simulink model "Control_try_2"  (R2021a)
settings: Solver=VariableStepAuto  StartTime=0.0  StopTime=inf  RelTol=1e-3
undefined symbols (not defined in the file or in its folder): DiscIntNeverNeededParam
libraries: mobileRoboticsLib x25
(part 1 of 2)
settings Model: Creator=its_ghani  LastModifiedBy=2737767G

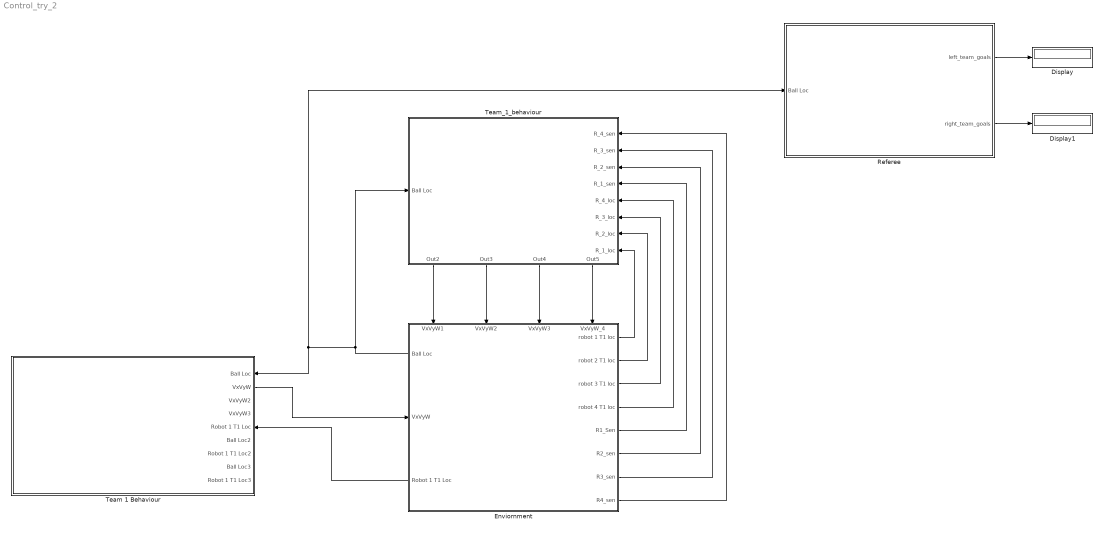
== system Control_try_2 ==
  Display : Display
  Display1 : Display
  Enviornment : Subsystem
      settings: PortSchema="{\"entries\":[{\"content\":{\"sides\":[{\"content\":{\"connectorIds\":[\"Out9\",\"In1\",\"Out10\"]},\"type\":\"ConnectorPlacement.EquallySpacedRectSide\",\"uuid\":\"bfc4f995-18bb-40a5-813e-439d500b4bf9\"},{\"content\":{\"connectorIds\":[\"Out1\",\"Out2\",\"Out3\",\"Out4\",\"Out5\",\"Out6\",\"Out7\",\"Out8\"],\"side\":\"RIGHT\"},\"type\":\"ConnectorPlacement.EquallySpacedRectSide\",\"uuid\":\"3fb6b8a6-16df-4a59-8ba5-6321e26d1fdd\"},{\"content\":{\"connectorIds\":[\"In2\",\"In3\",\"In4\",\"In5\"],\"side\":\"TOP\"},\"type\":\"ConnectorPlacement.EquallySpacedRectSide\",\"uuid\":\"a9e4cd1b-3afe-4395-99fa-15aef12a4070\"}]},\"type\":\"ConnectorPlacement.EquallySpacedConnector\",\"uuid\":\"a6ca697e-fe67-43ac-b669-91f3e6c836c9\"}],\"packageUris\":[\"http://schema.mathworks.com/mf0/Connector/R2020b\"],\"version\":\"1.0\"}"
  Referee : Subsystem
  Team 1 Behaviour : Subsystem
      settings: PortSchema="{\"entries\":[{\"content\":{\"sides\":[{\"content\":{\"connectorIds\":[]},\"type\":\"ConnectorPlacement.EquallySpacedRectSide\",\"uuid\":\"be901545-21b9-45e5-bac5-a8cb9027aef5\"},{\"content\":{\"connectorIds\":[\"In1\",\"Out1\",\"Out2\",\"Out3\",\"In2\",\"In3\",\"In4\",\"In5\",\"In6\"],\"side\":\"RIGHT\"},\"type\":\"ConnectorPlacement.EquallySpacedRectSide\",\"uuid\":\"b7c1eb84-2f14-4c7f-a74c-d56efbe0743e\"},{\"content\":{\"connectorIds\":[],\"side\":\"TOP\"},\"type\":\"ConnectorPlacement.EquallySpacedRectSide\",\"uuid\":\"aca41723-ed3f-4bd2-8fc1-457d075e3460\"}]},\"type\":\"ConnectorPlacement.EquallySpacedConnector\",\"uuid\":\"e10e22f1-c8f0-4dfc-85d2-4ba01528372d\"}],\"packageUris\":[\"http://schema.mathworks.com/mf0/Connector/R2020b\"],\"version\":\"1.0\"}"
  Team_1_behaviour : Subsystem
      settings: PortSchema="{\"entries\":[{\"content\":{\"sides\":[{\"content\":{\"connectorIds\":[\"In1\"]},\"type\":\"ConnectorPlacement.EquallySpacedRectSide\",\"uuid\":\"3d238569-03e8-47ba-93af-d09e13fdb2d4\"},{\"content\":{\"connectorIds\":[\"In2\",\"In3\",\"In4\",\"In5\",\"In6\",\"In7\",\"In8\",\"In9\"],\"side\":\"RIGHT\"},\"type\":\"ConnectorPlacement.EquallySpacedRectSide\",\"uuid\":\"12d8afb4-4727-4f82-8566-507ab080c6de\"},{\"content\":{\"connectorIds\":[],\"side\":\"TOP\"},\"type\":\"ConnectorPlacement.EquallySpacedRectSide\",\"uuid\":\"c52fa7ec-51b7-43be-84ca-6ce417c012c7\"},{\"content\":{\"connectorIds\":[\"Out1\",\"Out2\",\"Out3\",\"Out4\"],\"side\":\"BOTTOM\"},\"type\":\"ConnectorPlacement.EquallySpacedRectSide\",\"uuid\":\"1ba4ac49-8e90-4b3f-8374-c14756940453\"}]},\"type\":\"ConnectorPlacement.EquallySpacedConnector\",\"uuid\":\"883bb5df-d6b2-498f-94a4-3b94e28c6a8f\"}],\"packageUris\":[\"http://schema.mathworks.com/mf0/Connector/R2020b\"],\"version\":\"1.0\"}"
  wires:
  Enviornment/9(Ball Loc) -> Team_1_behaviour/1(Ball Loc), Referee/1(Ball Loc), Team 1 Behaviour/1(Ball Loc)
  Referee/2(right_team_goals) -> Display1/1
  Referee/1(left_team_goals) -> Display/1
  Team 1 Behaviour/1(VxVyW) -> Enviornment/1(VxVyW)
  Enviornment/10(Robot 1 T1 Loc) -> Team 1 Behaviour/2(Robot 1 T1 Loc)
  Team_1_behaviour/1(Out2) -> Enviornment/2(VxVyW1)
  Team_1_behaviour/2(Out3) -> Enviornment/3(VxVyW2)
  Team_1_behaviour/3(Out4) -> Enviornment/4(VxVyW3)
  Team_1_behaviour/4(Out5) -> Enviornment/5(VxVyW_4)
  Enviornment/1(robot 1 T1 loc) -> Team_1_behaviour/9(R_1_loc)
  Enviornment/2(robot 2 T1 loc) -> Team_1_behaviour/8(R_2_loc)
  Enviornment/3(robot 3 T1 loc) -> Team_1_behaviour/7(R_3_loc)
  Enviornment/4(robot 4 T1 loc) -> Team_1_behaviour/6(R_4_loc)
  Enviornment/5(R1_Sen) -> Team_1_behaviour/5(R_1_sen)
  Enviornment/6(R2_sen) -> Team_1_behaviour/4(R_2_sen)
  Enviornment/7(R3_sen) -> Team_1_behaviour/3(R_3_sen)
  Enviornment/8(R4_sen) -> Team_1_behaviour/2(R_4_sen)

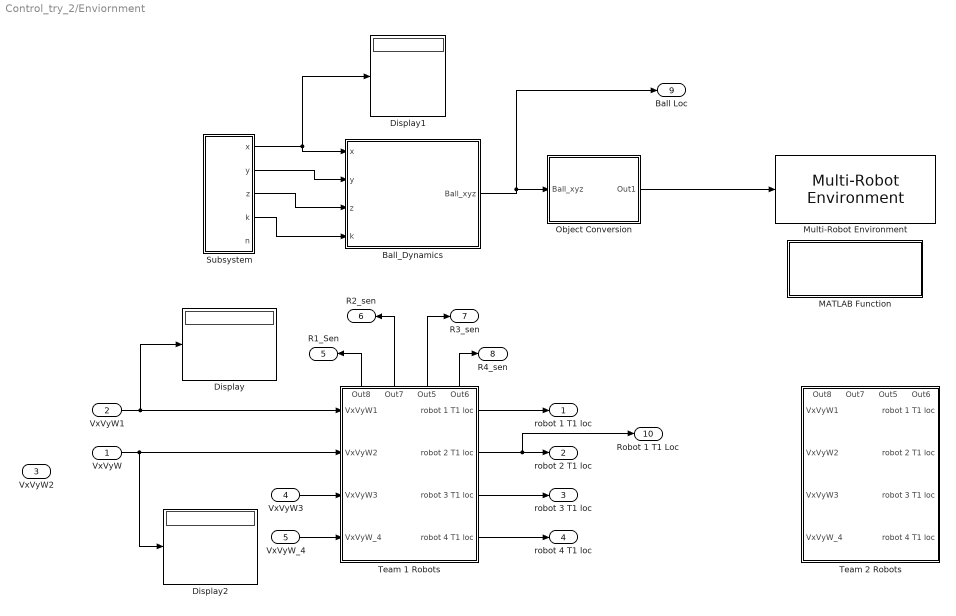
== system Control_try_2/Enviornment ==
  VxVyW : Inport
  VxVyW1 : Inport  Port=2
  VxVyW2 : Inport  Port=3
  VxVyW3 : Inport  Port=4
  VxVyW_4 : Inport  Port=5
  "\tTeam 1 Robots" : Subsystem
      settings: PortSchema="{\"entries\":[{\"content\":{\"sides\":[{\"content\":{\"connectorIds\":[\"In1\",\"In2\",\"In3\",\"In4\"]},\"type\":\"ConnectorPlacement.EquallySpacedRectSide\",\"uuid\":\"e759642f-fbca-4f1e-b212-daca2c4962f8\"},{\"content\":{\"connectorIds\":[\"Out1\",\"Out2\",\"Out3\",\"Out4\"],\"side\":\"RIGHT\"},\"type\":\"ConnectorPlacement.EquallySpacedRectSide\",\"uuid\":\"6e1699fa-b246-4758-836f-1d4c98857b70\"},{\"content\":{\"connectorIds\":[\"Out5\",\"Out6\",\"Out7\",\"Out8\"],\"side\":\"TOP\"},\"type\":\"ConnectorPlacement.EquallySpacedRectSide\",\"uuid\":\"c1cf0a96-808a-4241-9d01-181cc4ce2a4d\"},{\"content\":{\"connectorIds\":[],\"side\":\"BOTTOM\"},\"type\":\"ConnectorPlacement.EquallySpacedRectSide\",\"uuid\":\"1a7f648f-16d5-4a09-b479-d6590fa53252\"}]},\"type\":\"ConnectorPlacement.EquallySpacedConnector\",\"uuid\":\"5972ed04-ecdd-4117-bf5d-456318b5c4b8\"}],\"packageUris\":[\"http://schema.mathworks.com/mf0/Connector/R2020b\"],\"version\":\"1.0\"}"
  "\tTeam 2 Robots" : Subsystem
      settings: PortSchema="{\"entries\":[{\"content\":{\"sides\":[{\"content\":{\"connectorIds\":[\"In1\",\"In2\",\"In3\",\"In4\"]},\"type\":\"ConnectorPlacement.EquallySpacedRectSide\",\"uuid\":\"e759642f-fbca-4f1e-b212-daca2c4962f8\"},{\"content\":{\"connectorIds\":[\"Out1\",\"Out2\",\"Out3\",\"Out4\"],\"side\":\"RIGHT\"},\"type\":\"ConnectorPlacement.EquallySpacedRectSide\",\"uuid\":\"6e1699fa-b246-4758-836f-1d4c98857b70\"},{\"content\":{\"connectorIds\":[\"Out5\",\"Out6\",\"Out7\",\"Out8\"],\"side\":\"TOP\"},\"type\":\"ConnectorPlacement.EquallySpacedRectSide\",\"uuid\":\"c1cf0a96-808a-4241-9d01-181cc4ce2a4d\"},{\"content\":{\"connectorIds\":[],\"side\":\"BOTTOM\"},\"type\":\"ConnectorPlacement.EquallySpacedRectSide\",\"uuid\":\"1a7f648f-16d5-4a09-b479-d6590fa53252\"}]},\"type\":\"ConnectorPlacement.EquallySpacedConnector\",\"uuid\":\"5972ed04-ecdd-4117-bf5d-456318b5c4b8\"}],\"packageUris\":[\"http://schema.mathworks.com/mf0/Connector/R2020b\"],\"version\":\"1.0\"}"
  Ball_Dynamics : Subsystem
  Display : Display
  Display1 : Display
  Display2 : Display
  MATLAB Function : MATLAB Function  TreatAsAtomicUnit=on
  Multi-Robot Environment : mobileRoboticsLib/Environments/Multi-Robot Environment  numRobots=8  showWaypoints=off  showObjects=on  objectColors=[1 0 0;0 1 0;0 0 1]  objectMarkers='c'  showRobotIds=on  plotSensorLines=on
      settings: SourceProductName=Mobile Robotics Simulation Toolbox
  Object Conversion : Subsystem
  Subsystem : Subsystem
  robot 1 T1 loc : Outport
  robot 2 T1 loc : Outport  Port=2
  robot 3 T1 loc : Outport  Port=3
  robot 4 T1 loc : Outport  Port=4
  R1_Sen : Outport  Port=5
  R2_sen : Outport  Port=6
  R3_sen : Outport  Port=7
  R4_sen : Outport  Port=8
  Ball Loc : Outport  Port=9
  Robot 1 T1 Loc : Outport  Port=10
  wires:
  "\tTeam 1 Robots"/1(robot 1 T1 loc) -> robot 1 T1 loc/1
  Ball_Dynamics/1(Ball_xyz) -> Object Conversion/1(Ball_xyz), Ball Loc/1
  Object Conversion/1(Out1) -> Multi-Robot Environment/1
  "\tTeam 1 Robots"/2(robot 2 T1 loc) -> Robot 1 T1 Loc/1, robot 2 T1 loc/1
  "\tTeam 1 Robots"/3(robot 3 T1 loc) -> robot 3 T1 loc/1
  "\tTeam 1 Robots"/4(robot 4 T1 loc) -> robot 4 T1 loc/1
  VxVyW1/1 -> "\tTeam 1 Robots"/1(VxVyW1), Display/1
  VxVyW3/1 -> "\tTeam 1 Robots"/3(VxVyW3)
  VxVyW_4/1 -> "\tTeam 1 Robots"/4(VxVyW_4)
  "\tTeam 1 Robots"/5(Out8) -> R1_Sen/1
  "\tTeam 1 Robots"/6(Out7) -> R2_sen/1
  "\tTeam 1 Robots"/7(Out5) -> R3_sen/1
  "\tTeam 1 Robots"/8(Out6) -> R4_sen/1
  VxVyW/1 -> Display2/1, "\tTeam 1 Robots"/2(VxVyW2)
  Subsystem/1(x) -> Ball_Dynamics/1(x), Display1/1
  Subsystem/2(y) -> Ball_Dynamics/2(y)
  Subsystem/4(k) -> Ball_Dynamics/4(k)
  Subsystem/3(z) -> Ball_Dynamics/3(z)

== system Control_try_2/Referee ==
  Ball Loc : Inport
  Corner : Stateflow chart  TreatAsAtomicUnit=on
  Demux : Demux  Outputs=3
  Display2 : Display
  GOAL : Stateflow chart  TreatAsAtomicUnit=on
  Penelty : Stateflow chart  TreatAsAtomicUnit=on
  Throwin : Stateflow chart  TreatAsAtomicUnit=on
  left_team_goals : Outport
  right_team_goals : Outport  Port=2
  wires:
  Ball Loc/1 -> Display2/1, Demux/1
  Demux/1 -> Throwin/1(X), GOAL/1(X)
  Demux/2 -> Throwin/2(Y), GOAL/2(Y)
  Demux/3 -> GOAL/3(Z)
  GOAL/1(left_team_goal) -> left_team_goals/1
  GOAL/2(right_team_goal) -> right_team_goals/1

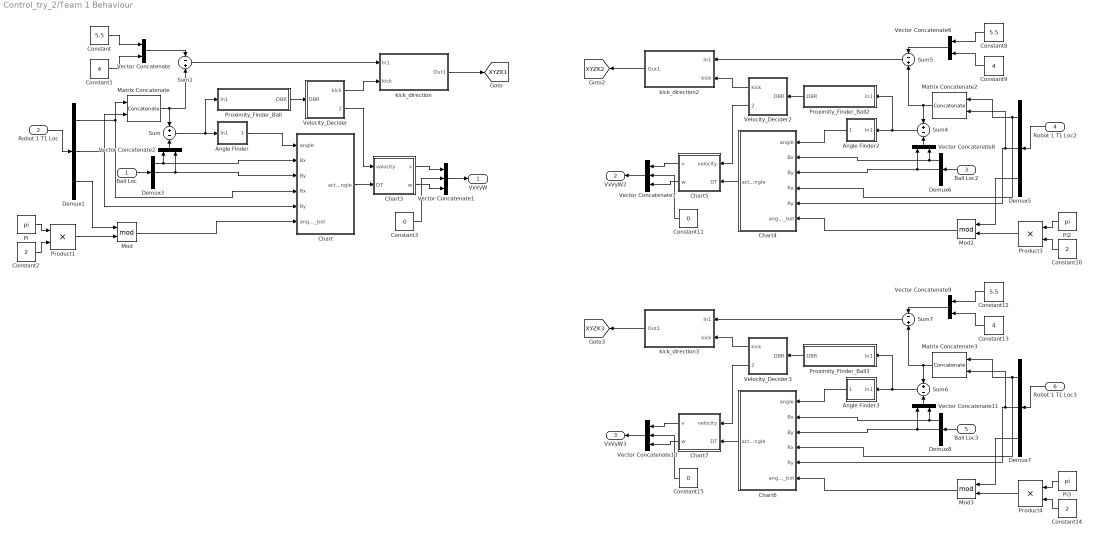
== system Control_try_2/Team 1 Behaviour ==
  Ball Loc : Inport
  Robot 1 T1 Loc : Inport  Port=2
  Ball Loc2 : Inport  Port=3
  Robot 1 T1 Loc2 : Inport  Port=4
  Ball Loc3 : Inport  Port=5
  Robot 1 T1 Loc3 : Inport  Port=6
  Angle Finder : Subsystem
  Angle Finder2 : Subsystem
  Angle Finder3 : Subsystem
  Chart : Stateflow chart  TreatAsAtomicUnit=on
      settings: PortSchema="{\"entries\":[{\"content\":{\"sides\":[{\"content\":{\"connectorIds\":[\"In5\",\"In1\",\"In2\",\"In3\",\"In4\",\"In6\"]},\"type\":\"ConnectorPlacement.EquallySpacedRectSide\",\"uuid\":\"cd25ea97-6441-4246-83f2-eec847899c89\"},{\"content\":{\"connectorIds\":[\"Out1\"],\"side\":\"RIGHT\"},\"type\":\"ConnectorPlacement.EquallySpacedRectSide\",\"uuid\":\"ef7d77a7-1549-4474-8b84-35bb8af5d0e7\"},{\"content\":{\"connectorIds\":[],\"side\":\"TOP\"},\"type\":\"ConnectorPlacement.EquallySpacedRectSide\",\"uuid\":\"0f0ce596-3061-42ac-890a-62bc4f21ac3e\"},{\"content\":{\"connectorIds\":[],\"side\":\"BOTTOM\"},\"type\":\"ConnectorPlacement.EquallySpacedRectSide\",\"uuid\":\"682b3de5-e999-4954-b7ff-f16ecbf9ea8f\"}]},\"type\":\"ConnectorPlacement.EquallySpacedConnector\",\"uuid\":\"15dca8e2-6a60-4a0d-80a5-3c295a61c828\"}],\"packageUris\":[\"http://schema.mathworks.com/mf0/Connector/R2020b\"],\"version\":\"1.0\"}"
  Chart3 : Stateflow chart  TreatAsAtomicUnit=on
  Chart4 : Stateflow chart  TreatAsAtomicUnit=on
      settings: PortSchema="{\"entries\":[{\"content\":{\"sides\":[{\"content\":{\"connectorIds\":[\"In5\",\"In1\",\"In2\",\"In3\",\"In4\",\"In6\"]},\"type\":\"ConnectorPlacement.EquallySpacedRectSide\",\"uuid\":\"cd25ea97-6441-4246-83f2-eec847899c89\"},{\"content\":{\"connectorIds\":[\"Out1\"],\"side\":\"RIGHT\"},\"type\":\"ConnectorPlacement.EquallySpacedRectSide\",\"uuid\":\"ef7d77a7-1549-4474-8b84-35bb8af5d0e7\"},{\"content\":{\"connectorIds\":[],\"side\":\"TOP\"},\"type\":\"ConnectorPlacement.EquallySpacedRectSide\",\"uuid\":\"0f0ce596-3061-42ac-890a-62bc4f21ac3e\"},{\"content\":{\"connectorIds\":[],\"side\":\"BOTTOM\"},\"type\":\"ConnectorPlacement.EquallySpacedRectSide\",\"uuid\":\"682b3de5-e999-4954-b7ff-f16ecbf9ea8f\"}]},\"type\":\"ConnectorPlacement.EquallySpacedConnector\",\"uuid\":\"15dca8e2-6a60-4a0d-80a5-3c295a61c828\"}],\"packageUris\":[\"http://schema.mathworks.com/mf0/Connector/R2020b\"],\"version\":\"1.0\"}"
  Chart5 : Stateflow chart  TreatAsAtomicUnit=on
  Chart6 : Stateflow chart  TreatAsAtomicUnit=on
      settings: PortSchema="{\"entries\":[{\"content\":{\"sides\":[{\"content\":{\"connectorIds\":[\"In5\",\"In1\",\"In2\",\"In3\",\"In4\",\"In6\"]},\"type\":\"ConnectorPlacement.EquallySpacedRectSide\",\"uuid\":\"cd25ea97-6441-4246-83f2-eec847899c89\"},{\"content\":{\"connectorIds\":[\"Out1\"],\"side\":\"RIGHT\"},\"type\":\"ConnectorPlacement.EquallySpacedRectSide\",\"uuid\":\"ef7d77a7-1549-4474-8b84-35bb8af5d0e7\"},{\"content\":{\"connectorIds\":[],\"side\":\"TOP\"},\"type\":\"ConnectorPlacement.EquallySpacedRectSide\",\"uuid\":\"0f0ce596-3061-42ac-890a-62bc4f21ac3e\"},{\"content\":{\"connectorIds\":[],\"side\":\"BOTTOM\"},\"type\":\"ConnectorPlacement.EquallySpacedRectSide\",\"uuid\":\"682b3de5-e999-4954-b7ff-f16ecbf9ea8f\"}]},\"type\":\"ConnectorPlacement.EquallySpacedConnector\",\"uuid\":\"15dca8e2-6a60-4a0d-80a5-3c295a61c828\"}],\"packageUris\":[\"http://schema.mathworks.com/mf0/Connector/R2020b\"],\"version\":\"1.0\"}"
  Chart7 : Stateflow chart  TreatAsAtomicUnit=on
  Constant : Constant  Value=5.5
  Constant1 : Constant  Value=4
  Constant10 : Constant  Value=2
  Constant11 : Constant  Value=0
  Constant12 : Constant  Value=5.5
  Constant13 : Constant  Value=4
  Constant14 : Constant  Value=2
  Constant15 : Constant  Value=0
  Constant2 : Constant  Value=2
  Constant3 : Constant  Value=0
  Constant8 : Constant  Value=5.5
  Constant9 : Constant  Value=4
  Demux{1,3,5..8} (6 alike) : Demux  Outputs=3
  Matrix Concatenate : Concatenate  Mode=Multidimensional array  ConcatenateDimension=2
  Matrix Concatenate2 : Concatenate  Mode=Multidimensional array  ConcatenateDimension=2
  Matrix Concatenate3 : Concatenate  Mode=Multidimensional array  ConcatenateDimension=2
  Mod : Math  Operator=mod  SaturateOnIntegerOverflow=on
  Mod2 : Math  Operator=mod  SaturateOnIntegerOverflow=on
  Mod3 : Math  Operator=mod  SaturateOnIntegerOverflow=on
  Pi : Constant  Value=pi  OutDataTypeStr=Inherit: Inherit via back propagation
  Pi2 : Constant  Value=pi  OutDataTypeStr=Inherit: Inherit via back propagation
  Pi3 : Constant  Value=pi  OutDataTypeStr=Inherit: Inherit via back propagation
  Product1 : Product
  Product3 : Product
  Product4 : Product
  Proximity_Finder_Ball : Subsystem
  Proximity_Finder_Ball2 : Subsystem
  Proximity_Finder_Ball3 : Subsystem
  Sum : Sum  Inputs=+-
  Sum1 : Sum  Inputs=-+
  Sum4 : Sum  Inputs=+-
  Sum5 : Sum  Inputs=-+
  Sum6 : Sum  Inputs=+-
  Sum7 : Sum  Inputs=-+
  Vector Concatenate{,2,6,8..9,11} (6 alike) : Concatenate
  Vector Concatenate1 : Concatenate  NumInputs=3
  Vector Concatenate10 : Concatenate  NumInputs=3
  Vector Concatenate7 : Concatenate  NumInputs=3
  Velocity_Decider : Stateflow chart  TreatAsAtomicUnit=on
  Velocity_Decider2 : Stateflow chart  TreatAsAtomicUnit=on
  Velocity_Decider3 : Stateflow chart  TreatAsAtomicUnit=on
  kick_direction : Subsystem
  kick_direction2 : Subsystem
  kick_direction3 : Subsystem
  VxVyW : Outport
  VxVyW2 : Outport  Port=2
  VxVyW3 : Outport  Port=3
  tag scope: XYZK1=global, XYZK2=global, XYZK3=global
  wires:
  Ball Loc/1 -> Demux3/1
  Sum/1 -> Proximity_Finder_Ball/1(In1), Angle Finder/1(In1)
  Robot 1 T1 Loc/1 -> Demux1/1
  Demux1/1 -> Matrix Concatenate/1, Chart/3(Rx)
  Demux1/2 -> Matrix Concatenate/2, Chart/4(Ry)
  Matrix Concatenate/1 -> Sum1/2, Sum/1
  Demux3/2 -> Vector Concatenate2/2, Chart/2(By)
  Demux3/1 -> Vector Concatenate2/1, Chart/1(Bx)
  Demux1/3 -> Mod/1
  Pi/1 -> Product1/1
  Constant2/1 -> Product1/2
  Product1/1 -> Mod/2
  Chart/1(actual_angle) -> Chart3/2(DT)
  Mod/1 -> Chart/6(angle_bot)
  Angle Finder/1(angle) -> Chart/5(angle)
  Proximity_Finder_Ball/1(DBR) -> Velocity_Decider/1(DBR)
  Velocity_Decider/2(velocity) -> Chart3/1(velocity)
  Constant/1 -> Vector Concatenate/1
  Constant1/1 -> Vector Concatenate/2
  Vector Concatenate/1 -> Sum1/1
  Sum1/1 -> kick_direction/1(In1)
  Velocity_Decider/1(kick) -> kick_direction/2(kick)
  kick_direction/1(Out1) -> [XYZK1]
  Chart3/1(v) -> Vector Concatenate1/1
  Chart3/2(w) -> Vector Concatenate1/3
  Constant3/1 -> Vector Concatenate1/2
  Vector Concatenate1/1 -> VxVyW/1
  Vector Concatenate2/1 -> Sum/2
  Constant11/1 -> Vector Concatenate7/2
  Pi2/1 -> Product3/1
  Chart5/1(v) -> Vector Concatenate7/1
  Vector Concatenate8/1 -> Sum4/2
  Velocity_Decider2/1(kick) -> kick_direction2/2(kick)
  Sum5/1 -> kick_direction2/1(In1)
  Velocity_Decider2/2(velocity) -> Chart5/1(velocity)
  Constant8/1 -> Vector Concatenate6/1
  Vector Concatenate7/1 -> VxVyW2/1
  Vector Concatenate6/1 -> Sum5/1
  Product3/1 -> Mod2/2
  Chart5/2(w) -> Vector Concatenate7/3
  Sum4/1 -> Proximity_Finder_Ball2/1(In1), Angle Finder2/1(In1)
  Constant10/1 -> Product3/2
  kick_direction2/1(Out1) -> [XYZK2]
  Demux6/2 -> Vector Concatenate8/2, Chart4/2(By)
  Chart4/1(actual_angle) -> Chart5/2(DT)
  Constant9/1 -> Vector Concatenate6/2
  Matrix Concatenate2/1 -> Sum5/2, Sum4/1
  Mod2/1 -> Chart4/6(angle_bot)
  Proximity_Finder_Ball2/1(DBR) -> Velocity_Decider2/1(DBR)
  Robot 1 T1 Loc2/1 -> Demux5/1
  Demux5/2 -> Matrix Concatenate2/2, Chart4/4(Ry)
  Demux5/1 -> Matrix Concatenate2/1, Chart4/3(Rx)
  Angle Finder2/1(angle) -> Chart4/5(angle)
  Demux6/1 -> Vector Concatenate8/1, Chart4/1(Bx)
  Ball Loc2/1 -> Demux6/1
  Demux5/3 -> Mod2/1
  Constant15/1 -> Vector Concatenate10/2
  Pi3/1 -> Product4/1
  Chart7/1(v) -> Vector Concatenate10/1
  Vector Concatenate11/1 -> Sum6/2
  Velocity_Decider3/1(kick) -> kick_direction3/2(kick)
  Sum7/1 -> kick_direction3/1(In1)
  Velocity_Decider3/2(velocity) -> Chart7/1(velocity)
  Constant12/1 -> Vector Concatenate9/1
  Vector Concatenate10/1 -> VxVyW3/1
  Vector Concatenate9/1 -> Sum7/1
  Product4/1 -> Mod3/2
  Chart7/2(w) -> Vector Concatenate10/3
  Sum6/1 -> Proximity_Finder_Ball3/1(In1), Angle Finder3/1(In1)
  Constant14/1 -> Product4/2
  kick_direction3/1(Out1) -> [XYZK3]
  Demux8/2 -> Vector Concatenate11/2, Chart6/2(By)
  Chart6/1(actual_angle) -> Chart7/2(DT)
  Constant13/1 -> Vector Concatenate9/2
  Matrix Concatenate3/1 -> Sum7/2, Sum6/1
  Mod3/1 -> Chart6/6(angle_bot)
  Proximity_Finder_Ball3/1(DBR) -> Velocity_Decider3/1(DBR)
  Robot 1 T1 Loc3/1 -> Demux7/1
  Demux7/2 -> Matrix Concatenate3/2, Chart6/4(Ry)
  Demux7/1 -> Matrix Concatenate3/1, Chart6/3(Rx)
  Angle Finder3/1(angle) -> Chart6/5(angle)
  Demux8/1 -> Vector Concatenate11/1, Chart6/1(Bx)
  Ball Loc3/1 -> Demux8/1
  Demux7/3 -> Mod3/1

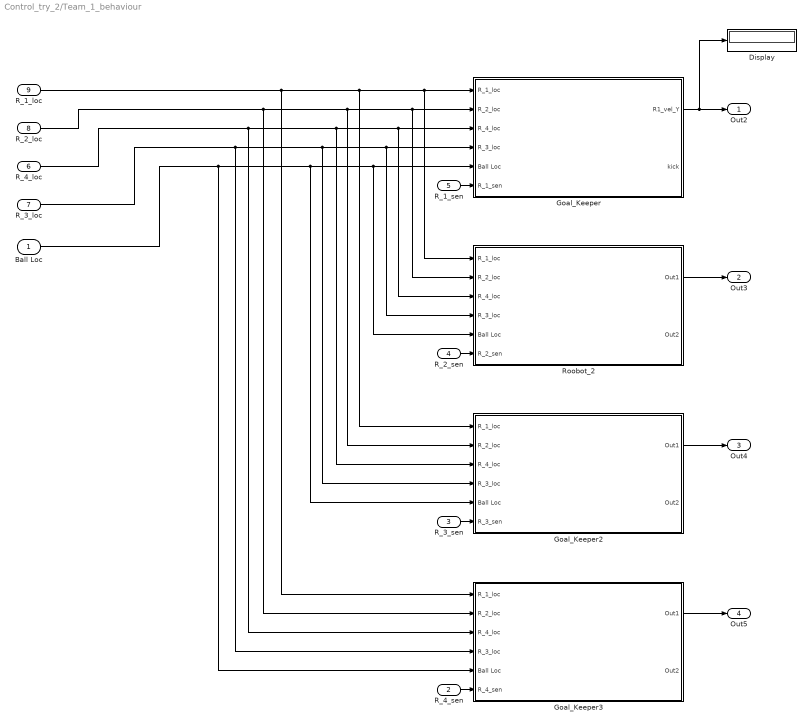
== system Control_try_2/Team_1_behaviour ==
  Ball Loc : Inport
  R_4_sen : Inport  Port=2
  R_3_sen : Inport  Port=3
  R_2_sen : Inport  Port=4
  R_1_sen : Inport  Port=5
  R_4_loc : Inport  Port=6
  R_3_loc : Inport  Port=7
  R_2_loc : Inport  Port=8
  R_1_loc : Inport  Port=9
  Display : Display
  Goal_Keeper : Subsystem
  Goal_Keeper2 : Subsystem
  Goal_Keeper3 : Subsystem
  Roobot_2 : Subsystem
  Out2 : Outport
  Out3 : Outport  Port=2
  Out4 : Outport  Port=3
  Out5 : Outport  Port=4
  wires:
  Goal_Keeper/1(R1_vel_Y) -> Display/1, Out2/1
  R_1_sen/1 -> Goal_Keeper/6(R_1_sen)
  R_1_loc/1 -> Goal_Keeper3/1(R_1_loc), Goal_Keeper2/1(R_1_loc), Roobot_2/1(R_1_loc), Goal_Keeper/1(R_1_loc)
  R_2_loc/1 -> Goal_Keeper3/2(R_2_loc), Goal_Keeper2/2(R_2_loc), Roobot_2/2(R_2_loc), Goal_Keeper/2(R_2_loc)
  R_4_loc/1 -> Goal_Keeper3/3(R_4_loc), Goal_Keeper2/3(R_4_loc), Roobot_2/3(R_4_loc), Goal_Keeper/3(R_4_loc)
  R_3_loc/1 -> Goal_Keeper3/4(R_3_loc), Goal_Keeper2/4(R_3_loc), Roobot_2/4(R_3_loc), Goal_Keeper/4(R_3_loc)
  Ball Loc/1 -> Goal_Keeper3/5(Ball Loc), Goal_Keeper2/5(Ball Loc), Roobot_2/5(Ball Loc), Goal_Keeper/5(Ball Loc)
  R_2_sen/1 -> Roobot_2/6(R_2_sen)
  R_3_sen/1 -> Goal_Keeper2/6(R_3_sen)
  R_4_sen/1 -> Goal_Keeper3/6(R_4_sen)
  Roobot_2/1(Out1) -> Out3/1
  Goal_Keeper2/1(Out1) -> Out4/1
  Goal_Keeper3/1(Out1) -> Out5/1

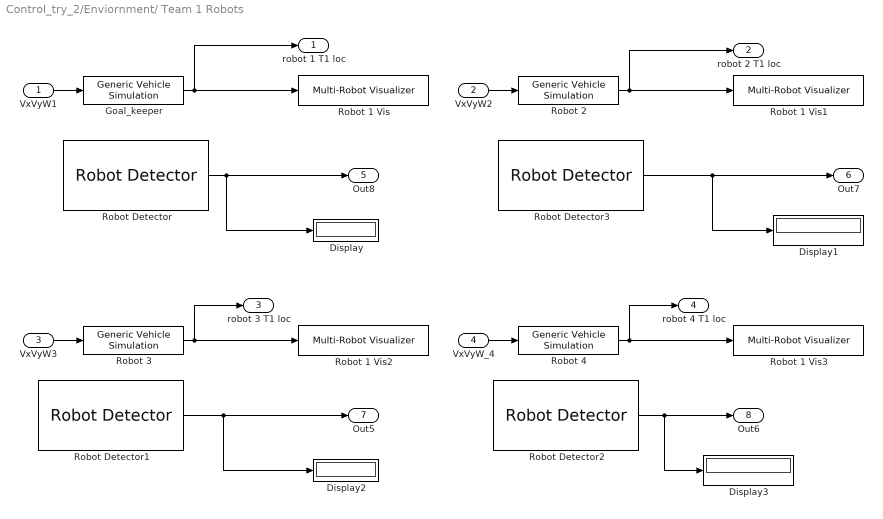
== system Control_try_2/Enviornment/	Team 1 Robots ==
  VxVyW1 : Inport
  VxVyW2 : Inport  Port=2
  VxVyW3 : Inport  Port=3
  VxVyW_4 : Inport  Port=4
  Display{,1..3} (4 alike) : Display
  Goal_keeper : mobileRoboticsLib/Utilities/Generic Vehicle Simulation  initX=1.5  initY=4  initAngle=0  Ts=0.05
      settings: SourceProductName=Mobile Robotics Simulation Toolbox
  Robot 1 Vis : mobileRoboticsLib/Environments/Multi-Robot Visualizer  idx=1  radius=0.5  robotColor=[0 0 1]  showTraj=on  hasLidar=off  sensorOffset=[0,0]  scanAngles=[-pi/4, 0, pi/4]  maxNumScans=0  hasObjDetector=off  objDetectorOffset=[0,0]  objDetectorAngle=0  objDetectorFOV=pi/3  objDetectorMaxRange=5  hasRobotDetector=off  robotDetectorOffset=[0,0]  robotDetectorAngle=0  robotDetectorFOV=pi/3  robotDetectorMaxRange=5  robotDetectorNumDetections=0
      settings: SourceProductName=Mobile Robotics Simulation Toolbox
  Robot 1 Vis1 : mobileRoboticsLib/Environments/Multi-Robot Visualizer  idx=2  radius=0.5  robotColor=[0 0 1]  showTraj=on  hasLidar=off  sensorOffset=[0,0]  scanAngles=[-pi/4, 0, pi/4]  maxNumScans=0  hasObjDetector=off  objDetectorOffset=[0,0]  objDetectorAngle=0  objDetectorFOV=pi/3  objDetectorMaxRange=5  hasRobotDetector=off  robotDetectorOffset=[0,0]  robotDetectorAngle=0  robotDetectorFOV=pi/3  robotDetectorMaxRange=5  robotDetectorNumDetections=0
      settings: SourceProductName=Mobile Robotics Simulation Toolbox
  Robot 1 Vis2 : mobileRoboticsLib/Environments/Multi-Robot Visualizer  idx=3  radius=0.5  robotColor=[0 0 1]  showTraj=on  hasLidar=off  sensorOffset=[0,0]  scanAngles=[-pi/4, 0, pi/4]  maxNumScans=0  hasObjDetector=off  objDetectorOffset=[0,0]  objDetectorAngle=0  objDetectorFOV=pi/3  objDetectorMaxRange=5  hasRobotDetector=off  robotDetectorOffset=[0,0]  robotDetectorAngle=0  robotDetectorFOV=pi/3  robotDetectorMaxRange=5  robotDetectorNumDetections=0
      settings: SourceProductName=Mobile Robotics Simulation Toolbox
  Robot 1 Vis3 : mobileRoboticsLib/Environments/Multi-Robot Visualizer  idx=4  radius=0.5  robotColor=[0 0 1]  showTraj=on  hasLidar=off  sensorOffset=[0,0]  scanAngles=[-pi/4, 0, pi/4]  maxNumScans=0  hasObjDetector=off  objDetectorOffset=[0,0]  objDetectorAngle=0  objDetectorFOV=pi/3  objDetectorMaxRange=5  hasRobotDetector=off  robotDetectorOffset=[0,0]  robotDetectorAngle=0  robotDetectorFOV=pi/3  robotDetectorMaxRange=5  robotDetectorNumDetections=0
      settings: SourceProductName=Mobile Robotics Simulation Toolbox
  Robot 2 : mobileRoboticsLib/Utilities/Generic Vehicle Simulation  initX=3.25  initY=2.5  initAngle=0  Ts=0.05
      settings: SourceProductName=Mobile Robotics Simulation Toolbox
  Robot 3 : mobileRoboticsLib/Utilities/Generic Vehicle Simulation  initX=3.25  initY=5.5  initAngle=0  Ts=0.05
      settings: SourceProductName=Mobile Robotics Simulation Toolbox
  Robot 4 : mobileRoboticsLib/Utilities/Generic Vehicle Simulation  initX=5.25  initY=4.25  initAngle=0  Ts=0.05
      settings: SourceProductName=Mobile Robotics Simulation Toolbox
  Robot Detector : mobileRoboticsLib/Environments/Robot Detector  mapName=map  robotIdx=1  sensorOffset=[ 0, 0 ]  sensorAngle=0  sensorFOV=pi/3  maxRange=3  maxDetections=7  sampleTime=0.1
      settings: SourceProductName=Mobile Robotics Simulation Toolbox
  Robot Detector1 : mobileRoboticsLib/Environments/Robot Detector  mapName=map  robotIdx=3  sensorOffset=[ 0, 0 ]  sensorAngle=0  sensorFOV=pi/3  maxRange=1.5  maxDetections=7  sampleTime=0.1
      settings: SourceProductName=Mobile Robotics Simulation Toolbox
  Robot Detector2 : mobileRoboticsLib/Environments/Robot Detector  mapName=map  robotIdx=4  sensorOffset=[ 0, 0 ]  sensorAngle=0  sensorFOV=pi/3  maxRange=1.5  maxDetections=7  sampleTime=0.1
      settings: SourceProductName=Mobile Robotics Simulation Toolbox
  Robot Detector3 : mobileRoboticsLib/Environments/Robot Detector  mapName=map  robotIdx=2  sensorOffset=[ 0, 0 ]  sensorAngle=0  sensorFOV=pi/3  maxRange=1.5  maxDetections=7  sampleTime=0.1
      settings: SourceProductName=Mobile Robotics Simulation Toolbox
  robot 1 T1 loc : Outport
  robot 2 T1 loc : Outport  Port=2
  robot 3 T1 loc : Outport  Port=3
  robot 4 T1 loc : Outport  Port=4
  Out8 : Outport  Port=5
  Out7 : Outport  Port=6
  Out5 : Outport  Port=7
  Out6 : Outport  Port=8
  wires:
  Goal_keeper/1 -> robot 1 T1 loc/1, Robot 1 Vis/1
  VxVyW1/1 -> Goal_keeper/1
  VxVyW2/1 -> Robot 2/1
  Robot 2/1 -> robot 2 T1 loc/1, Robot 1 Vis1/1
  Robot 3/1 -> Robot 1 Vis2/1, robot 3 T1 loc/1
  VxVyW3/1 -> Robot 3/1
  VxVyW_4/1 -> Robot 4/1
  Robot 4/1 -> robot 4 T1 loc/1, Robot 1 Vis3/1
  Robot Detector3/1 -> Out7/1, Display1/1
  Robot Detector1/1 -> Out5/1, Display2/1
  Robot Detector2/1 -> Out6/1, Display3/1
  Robot Detector/1 -> Display/1, Out8/1

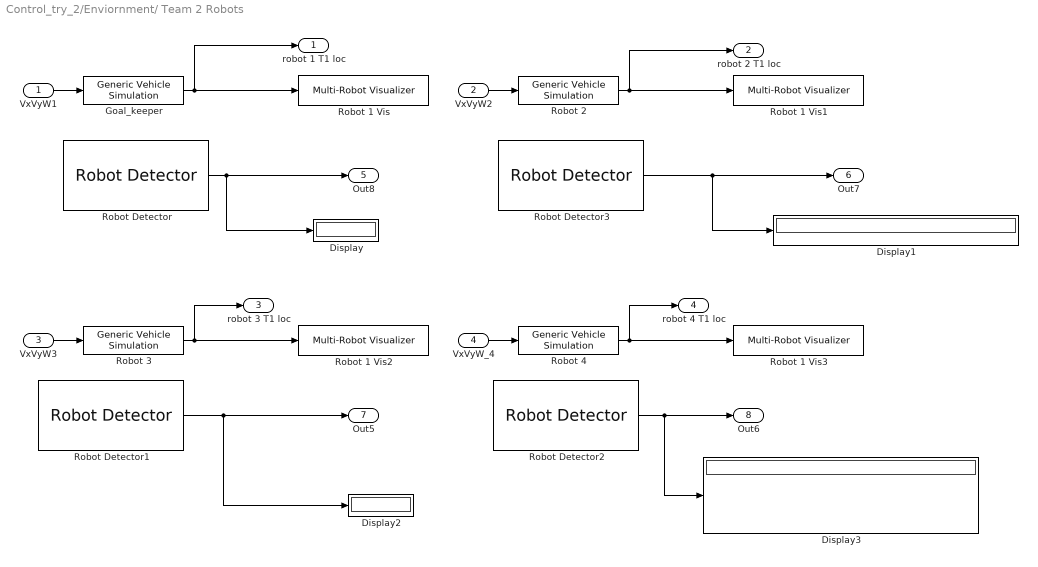
== system Control_try_2/Enviornment/	Team 2 Robots ==
  VxVyW1 : Inport
  VxVyW2 : Inport  Port=2
  VxVyW3 : Inport  Port=3
  VxVyW_4 : Inport  Port=4
  Display{,1..3} (4 alike) : Display
  Goal_keeper : mobileRoboticsLib/Utilities/Generic Vehicle Simulation  initX=9.5  initY=4  initAngle=pi  Ts=0.05
      settings: SourceProductName=Mobile Robotics Simulation Toolbox
  Robot 1 Vis : mobileRoboticsLib/Environments/Multi-Robot Visualizer  idx=5  radius=0.5  robotColor=[1 0 0]  showTraj=on  hasLidar=off  sensorOffset=[0,0]  scanAngles=[-pi/4, 0, pi/4]  maxNumScans=0  hasObjDetector=off  objDetectorOffset=[0,0]  objDetectorAngle=0  objDetectorFOV=pi/3  objDetectorMaxRange=5  hasRobotDetector=off  robotDetectorOffset=[0,0]  robotDetectorAngle=0  robotDetectorFOV=pi/3  robotDetectorMaxRange=5  robotDetectorNumDetections=0
      settings: SourceProductName=Mobile Robotics Simulation Toolbox
  Robot 1 Vis1 : mobileRoboticsLib/Environments/Multi-Robot Visualizer  idx=6  radius=0.5  robotColor=[0.1 1 1]  showTraj=on  hasLidar=off  sensorOffset=[0,0]  scanAngles=[-pi/4, 0, pi/4]  maxNumScans=0  hasObjDetector=off  objDetectorOffset=[0,0]  objDetectorAngle=0  objDetectorFOV=pi/3  objDetectorMaxRange=5  hasRobotDetector=off  robotDetectorOffset=[0,0]  robotDetectorAngle=0  robotDetectorFOV=pi/3  robotDetectorMaxRange=5  robotDetectorNumDetections=0
      settings: SourceProductName=Mobile Robotics Simulation Toolbox
  Robot 1 Vis2 : mobileRoboticsLib/Environments/Multi-Robot Visualizer  idx=7  radius=0.5  robotColor=[0 1 1]  showTraj=on  hasLidar=off  sensorOffset=[0,0]  scanAngles=[-pi/4, 0, pi/4]  maxNumScans=0  hasObjDetector=off  objDetectorOffset=[0,0]  objDetectorAngle=0  objDetectorFOV=pi/3  objDetectorMaxRange=5  hasRobotDetector=off  robotDetectorOffset=[0,0]  robotDetectorAngle=0  robotDetectorFOV=pi/3  robotDetectorMaxRange=5  robotDetectorNumDetections=0
      settings: SourceProductName=Mobile Robotics Simulation Toolbox
  Robot 1 Vis3 : mobileRoboticsLib/Environments/Multi-Robot Visualizer  idx=8  radius=0.5  robotColor=[0 1 1]  showTraj=on  hasLidar=off  sensorOffset=[0,0]  scanAngles=[-pi/4, 0, pi/4]  maxNumScans=0  hasObjDetector=off  objDetectorOffset=[0,0]  objDetectorAngle=0  objDetectorFOV=pi/3  objDetectorMaxRange=5  hasRobotDetector=off  robotDetectorOffset=[0,0]  robotDetectorAngle=0  robotDetectorFOV=pi/3  robotDetectorMaxRange=5  robotDetectorNumDetections=0
      settings: SourceProductName=Mobile Robotics Simulation Toolbox
  Robot 2 : mobileRoboticsLib/Utilities/Generic Vehicle Simulation  initX=3.5  initY=4  initAngle=pi  Ts=0.05
      settings: SourceProductName=Mobile Robotics Simulation Toolbox
  Robot 3 : mobileRoboticsLib/Utilities/Generic Vehicle Simulation  initX=3.5  initY=3  initAngle=pi  Ts=0.05
      settings: SourceProductName=Mobile Robotics Simulation Toolbox
  Robot 4 : mobileRoboticsLib/Utilities/Generic Vehicle Simulation  initX=7.75  initY=2.5  initAngle=pi  Ts=0.05
      settings: SourceProductName=Mobile Robotics Simulation Toolbox
  Robot Detector : mobileRoboticsLib/Environments/Robot Detector  mapName=map  robotIdx=5  sensorOffset=[ 0, 0 ]  sensorAngle=0  sensorFOV=pi/3  maxRange=1.5  maxDetections=7  sampleTime=0.1
      settings: SourceProductName=Mobile Robotics Simulation Toolbox
  Robot Detector1 : mobileRoboticsLib/Environments/Robot Detector  mapName=map  robotIdx=7  sensorOffset=[ 0, 0 ]  sensorAngle=0  sensorFOV=pi/3  maxRange=1.5  maxDetections=7  sampleTime=0.1
      settings: SourceProductName=Mobile Robotics Simulation Toolbox
  Robot Detector2 : mobileRoboticsLib/Environments/Robot Detector  mapName=map  robotIdx=8  sensorOffset=[ 0, 0 ]  sensorAngle=0  sensorFOV=pi/3  maxRange=1.5  maxDetections=7  sampleTime=0.1
      settings: SourceProductName=Mobile Robotics Simulation Toolbox
  Robot Detector3 : mobileRoboticsLib/Environments/Robot Detector  mapName=map  robotIdx=6  sensorOffset=[ 0, 0 ]  sensorAngle=0  sensorFOV=pi/3  maxRange=1.5  maxDetections=7  sampleTime=0.1
      settings: SourceProductName=Mobile Robotics Simulation Toolbox
  robot 1 T1 loc : Outport
  robot 2 T1 loc : Outport  Port=2
  robot 3 T1 loc : Outport  Port=3
  robot 4 T1 loc : Outport  Port=4
  Out8 : Outport  Port=5
  Out7 : Outport  Port=6
  Out5 : Outport  Port=7
  Out6 : Outport  Port=8
  wires:
  Goal_keeper/1 -> robot 1 T1 loc/1, Robot 1 Vis/1
  VxVyW1/1 -> Goal_keeper/1
  VxVyW2/1 -> Robot 2/1
  Robot 2/1 -> robot 2 T1 loc/1, Robot 1 Vis1/1
  Robot 3/1 -> Robot 1 Vis2/1, robot 3 T1 loc/1
  VxVyW3/1 -> Robot 3/1
  VxVyW_4/1 -> Robot 4/1
  Robot 4/1 -> robot 4 T1 loc/1, Robot 1 Vis3/1
  Robot Detector3/1 -> Out7/1, Display1/1
  Robot Detector1/1 -> Out5/1, Display2/1
  Robot Detector2/1 -> Out6/1, Display3/1
  Robot Detector/1 -> Display/1, Out8/1

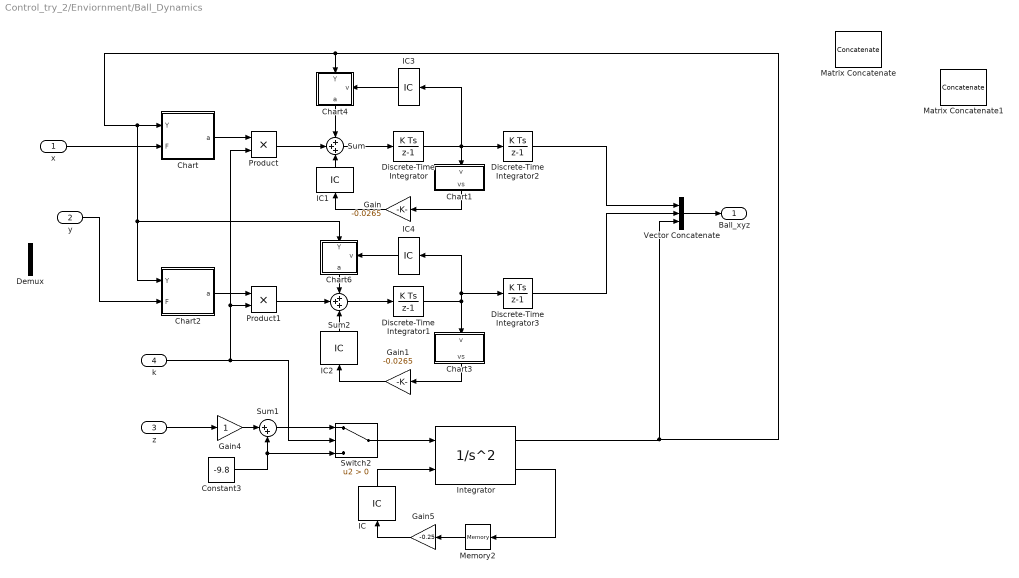
== system Control_try_2/Enviornment/Ball_Dynamics ==
  x : Inport
  y : Inport  Port=2
  z : Inport  Port=3
  k : Inport  Port=4
  Chart : Stateflow chart  TreatAsAtomicUnit=on
  Chart1 : Stateflow chart  TreatAsAtomicUnit=on
      settings: PortSchema="{\"entries\":[{\"content\":{\"sides\":[{\"content\":{\"connectorIds\":[]},\"type\":\"ConnectorPlacement.EquallySpacedRectSide\",\"uuid\":\"edcb69b6-c92b-474e-86d7-1e52c2e82b28\"},{\"content\":{\"connectorIds\":[],\"side\":\"RIGHT\"},\"type\":\"ConnectorPlacement.EquallySpacedRectSide\",\"uuid\":\"df9771e4-6870-4305-9c84-3f71fcb76e6b\"},{\"content\":{\"connectorIds\":[\"In1\"],\"side\":\"TOP\"},\"type\":\"ConnectorPlacement.EquallySpacedRectSide\",\"uuid\":\"56b80241-156d-4669-9174-884a577f2013\"},{\"content\":{\"connectorIds\":[\"Out1\"],\"side\":\"BOTTOM\"},\"type\":\"ConnectorPlacement.EquallySpacedRectSide\",\"uuid\":\"179af6a7-cab5-4faa-a562-268e2d2e4d3e\"}]},\"type\":\"ConnectorPlacement.EquallySpacedConnector\",\"uuid\":\"707001f1-02b8-4f5e-ba3f-f155c99072e5\"}],\"packageUris\":[\"http://schema.mathworks.com/mf0/Connector/R2020b\"],\"version\":\"1.0\"}"
  Chart2 : Stateflow chart  TreatAsAtomicUnit=on
  Chart3 : Stateflow chart  TreatAsAtomicUnit=on
      settings: PortSchema="{\"entries\":[{\"content\":{\"sides\":[{\"content\":{\"connectorIds\":[]},\"type\":\"ConnectorPlacement.EquallySpacedRectSide\",\"uuid\":\"edcb69b6-c92b-474e-86d7-1e52c2e82b28\"},{\"content\":{\"connectorIds\":[],\"side\":\"RIGHT\"},\"type\":\"ConnectorPlacement.EquallySpacedRectSide\",\"uuid\":\"df9771e4-6870-4305-9c84-3f71fcb76e6b\"},{\"content\":{\"connectorIds\":[\"In1\"],\"side\":\"TOP\"},\"type\":\"ConnectorPlacement.EquallySpacedRectSide\",\"uuid\":\"56b80241-156d-4669-9174-884a577f2013\"},{\"content\":{\"connectorIds\":[\"Out1\"],\"side\":\"BOTTOM\"},\"type\":\"ConnectorPlacement.EquallySpacedRectSide\",\"uuid\":\"179af6a7-cab5-4faa-a562-268e2d2e4d3e\"}]},\"type\":\"ConnectorPlacement.EquallySpacedConnector\",\"uuid\":\"707001f1-02b8-4f5e-ba3f-f155c99072e5\"}],\"packageUris\":[\"http://schema.mathworks.com/mf0/Connector/R2020b\"],\"version\":\"1.0\"}"
  Chart4 : Stateflow chart  TreatAsAtomicUnit=on
      settings: PortSchema="{\"entries\":[{\"content\":{\"sides\":[{\"content\":{\"connectorIds\":[]},\"type\":\"ConnectorPlacement.EquallySpacedRectSide\",\"uuid\":\"edcb69b6-c92b-474e-86d7-1e52c2e82b28\"},{\"content\":{\"connectorIds\":[\"In2\"],\"side\":\"RIGHT\"},\"type\":\"ConnectorPlacement.EquallySpacedRectSide\",\"uuid\":\"df9771e4-6870-4305-9c84-3f71fcb76e6b\"},{\"content\":{\"connectorIds\":[\"In1\"],\"side\":\"TOP\"},\"type\":\"ConnectorPlacement.EquallySpacedRectSide\",\"uuid\":\"56b80241-156d-4669-9174-884a577f2013\"},{\"content\":{\"connectorIds\":[\"Out1\"],\"side\":\"BOTTOM\"},\"type\":\"ConnectorPlacement.EquallySpacedRectSide\",\"uuid\":\"6d9abc99-74e1-40c2-a49f-e0d9410a29cc\"}]},\"type\":\"ConnectorPlacement.EquallySpacedConnector\",\"uuid\":\"707001f1-02b8-4f5e-ba3f-f155c99072e5\"}],\"packageUris\":[\"http://schema.mathworks.com/mf0/Connector/R2020b\"],\"version\":\"1.0\"}"
  Chart6 : Stateflow chart  TreatAsAtomicUnit=on
      settings: PortSchema="{\"entries\":[{\"content\":{\"sides\":[{\"content\":{\"connectorIds\":[]},\"type\":\"ConnectorPlacement.EquallySpacedRectSide\",\"uuid\":\"edcb69b6-c92b-474e-86d7-1e52c2e82b28\"},{\"content\":{\"connectorIds\":[\"In2\"],\"side\":\"RIGHT\"},\"type\":\"ConnectorPlacement.EquallySpacedRectSide\",\"uuid\":\"df9771e4-6870-4305-9c84-3f71fcb76e6b\"},{\"content\":{\"connectorIds\":[\"In1\"],\"side\":\"TOP\"},\"type\":\"ConnectorPlacement.EquallySpacedRectSide\",\"uuid\":\"56b80241-156d-4669-9174-884a577f2013\"},{\"content\":{\"connectorIds\":[\"Out1\"],\"side\":\"BOTTOM\"},\"type\":\"ConnectorPlacement.EquallySpacedRectSide\",\"uuid\":\"6d9abc99-74e1-40c2-a49f-e0d9410a29cc\"}]},\"type\":\"ConnectorPlacement.EquallySpacedConnector\",\"uuid\":\"707001f1-02b8-4f5e-ba3f-f155c99072e5\"}],\"packageUris\":[\"http://schema.mathworks.com/mf0/Connector/R2020b\"],\"version\":\"1.0\"}"
  Constant3 : Constant  Value=-9.8
  Demux : Demux
  Discrete-Time Integrator : DiscreteIntegrator  SampleTime=-1  ICPrevOutput=DiscIntNeverNeededParam  ICPrevScaledInput=DiscIntNeverNeededParam
  Discrete-Time Integrator1 : DiscreteIntegrator  SampleTime=-1  ICPrevOutput=DiscIntNeverNeededParam  ICPrevScaledInput=DiscIntNeverNeededParam
  Discrete-Time Integrator2 : DiscreteIntegrator  InitialCondition=5.5  SampleTime=-1  ICPrevOutput=DiscIntNeverNeededParam  ICPrevScaledInput=DiscIntNeverNeededParam
  Discrete-Time Integrator3 : DiscreteIntegrator  InitialCondition=7  SampleTime=-1  ICPrevOutput=DiscIntNeverNeededParam  ICPrevScaledInput=DiscIntNeverNeededParam
  Gain : Gain  Gain=-0.0265
  Gain1 : Gain  Gain=-0.0265
  Gain4 : Gain
  Gain5 : Gain  Gain=-0.25
  IC : InitialCondition
  IC{1..4} (4 alike) : InitialCondition  Value=0
  Integrator : SecondOrderIntegrator  ICX=0  LimitX=on  LowerLimitX=0.0  StateNameX='Position'  ICSourceDXDT=external  StateNameDXDT='Velocity'  ReinitDXDTwhenXreachesSaturation=on
  Matrix Concatenate : Concatenate  Mode=Multidimensional array  ConcatenateDimension=2
  Matrix Concatenate1 : Concatenate  Mode=Multidimensional array  ConcatenateDimension=2
  Memory2 : Memory
  Product : Product
  Product1 : Product
  Sum : Sum  Inputs=+++
  Sum1 : Sum  Inputs=|++
  Sum2 : Sum  Inputs=+++
  Switch2 : Switch  Criteria=u2 > Threshold
  Vector Concatenate : Concatenate  NumInputs=3
  Ball_xyz : Outport
  wires:
  Constant3/1 -> Sum1/2, Switch2/3
  Integrator/2 -> Memory2/1
  Memory2/1 -> Gain5/1
  IC/1 -> Integrator/2
  Switch2/1 -> Integrator/1
  Sum1/1 -> Switch2/1
  Gain4/1 -> Sum1/1
  z/1 -> Gain4/1
  k/1 -> Product/2, Product1/2, Switch2/2
  Gain5/1 -> IC/1
  Gain/1 -> IC1/1
  Chart/1(a) -> Product/1
  Sum/1 -> Discrete-Time Integrator/1
  Discrete-Time Integrator1/1 -> IC4/1, Discrete-Time Integrator3/1, Chart3/1(v)
  Chart2/1(a) -> Product1/1
  Gain1/1 -> IC2/1
  Product1/1 -> Sum2/2
  Sum2/1 -> Discrete-Time Integrator1/1
  x/1 -> Chart/2(F)
  y/1 -> Chart2/2(F)
  Integrator/1 -> Vector Concatenate/3, Chart6/1(Y), Chart2/1(Y), Chart/1(Y), Chart4/1(Y)
  Chart1/1(vs) -> Gain/1
  Chart3/1(vs) -> Gain1/1
  IC3/1 -> Chart4/2(v)
  Discrete-Time Integrator/1 -> IC3/1, Discrete-Time Integrator2/1, Chart1/1(v)
  Product/1 -> Sum/2
  IC2/1 -> Sum2/3
  IC1/1 -> Sum/3
  IC4/1 -> Chart6/2(v)
  Chart4/1(a) -> Sum/1
  Chart6/1(a) -> Sum2/1
  Vector Concatenate/1 -> Ball_xyz/1
  Discrete-Time Integrator2/1 -> Vector Concatenate/1
  Discrete-Time Integrator3/1 -> Vector Concatenate/2

== system Control_try_2/Enviornment/Object Conversion ==
  Ball_xyz : Inport
  Ball : Constant
  Demux : Demux  Outputs=3
  Matrix Concatenate : Concatenate  NumInputs=3  Mode=Multidimensional array  ConcatenateDimension=2
  Out1 : Outport
  wires:
  Ball/1 -> Matrix Concatenate/3
  Matrix Concatenate/1 -> Out1/1
  Ball_xyz/1 -> Demux/1
  Demux/1 -> Matrix Concatenate/1
  Demux/2 -> Matrix Concatenate/2

== system Control_try_2/Enviornment/Subsystem ==
  Demux : Demux
  Demux1 : Demux
  Demux2 : Demux
  MATLAB Function : MATLAB Function  TreatAsAtomicUnit=on
  x : Outport
  y : Outport  Port=2
  z : Outport  Port=3
  k : Outport  Port=4
  n : Outport  Port=5
  wires:
  [XYZK1] -> Demux/1
  [XYZK2] -> Demux1/1
  [XYZK3] -> Demux2/1
  Demux/1 -> MATLAB Function/1(x1)
  Demux/4 -> MATLAB Function/4(k1)
  Demux/3 -> MATLAB Function/3(z1)
  Demux/2 -> MATLAB Function/2(y1)
  MATLAB Function/1(x) -> x/1
  MATLAB Function/2(y) -> y/1
  MATLAB Function/3(z) -> z/1
  MATLAB Function/4(k) -> k/1
  Demux1/1 -> MATLAB Function/5(x2)
  Demux1/2 -> MATLAB Function/6(y2)
  Demux1/3 -> MATLAB Function/7(z2)
  Demux1/4 -> MATLAB Function/8(k2)
  Demux2/4 -> MATLAB Function/12(k3)
  Demux2/3 -> MATLAB Function/11(z3)
  Demux2/2 -> MATLAB Function/10(y3)
  Demux2/1 -> MATLAB Function/9(x3)
  MATLAB Function/5(n) -> n/1

== system Control_try_2/Team 1 Behaviour/Angle Finder ==
  In1 : Inport
  Abs : Abs
  Atan : Trigonometry  Operator=atan
  Demux : Demux  Outputs=2
  Divide : Product  Inputs=/*
  angle : Outport
  wires:
  Divide/1 -> Atan/1
  Demux/2 -> Divide/2
  Demux/1 -> Divide/1
  Atan/1 -> Abs/1
  Abs/1 -> angle/1
  In1/1 -> Demux/1

== system Control_try_2/Team 1 Behaviour/Angle Finder2 ==
  In1 : Inport
  Abs : Abs
  Atan : Trigonometry  Operator=atan
  Demux : Demux  Outputs=2
  Divide : Product  Inputs=/*
  angle : Outport
  wires:
  Divide/1 -> Atan/1
  Demux/2 -> Divide/2
  Demux/1 -> Divide/1
  Atan/1 -> Abs/1
  Abs/1 -> angle/1
  In1/1 -> Demux/1

== system Control_try_2/Team 1 Behaviour/Angle Finder3 ==
  In1 : Inport
  Abs : Abs
  Atan : Trigonometry  Operator=atan
  Demux : Demux  Outputs=2
  Divide : Product  Inputs=/*
  angle : Outport
  wires:
  Divide/1 -> Atan/1
  Demux/2 -> Divide/2
  Demux/1 -> Divide/1
  Atan/1 -> Abs/1
  Abs/1 -> angle/1
  In1/1 -> Demux/1

== system Control_try_2/Team 1 Behaviour/Proximity_Finder_Ball ==
  In1 : Inport
  Demux : Demux  Outputs=2
  Sqrt : Sqrt  SaturateOnIntegerOverflow=on
  Square : Math  Operator=square  SaturateOnIntegerOverflow=on
  Square1 : Math  Operator=square  SaturateOnIntegerOverflow=on
  Sum : Sum
  DBR : Outport
  wires:
  In1/1 -> Demux/1
  Demux/1 -> Square/1
  Demux/2 -> Square1/1
  Square1/1 -> Sum/2
  Square/1 -> Sum/1
  Sum/1 -> Sqrt/1
  Sqrt/1 -> DBR/1

== system Control_try_2/Team 1 Behaviour/Proximity_Finder_Ball2 ==
  In1 : Inport
  Demux : Demux  Outputs=2
  Sqrt : Sqrt  SaturateOnIntegerOverflow=on
  Square : Math  Operator=square  SaturateOnIntegerOverflow=on
  Square1 : Math  Operator=square  SaturateOnIntegerOverflow=on
  Sum : Sum
  DBR : Outport
  wires:
  In1/1 -> Demux/1
  Demux/1 -> Square/1
  Demux/2 -> Square1/1
  Square1/1 -> Sum/2
  Square/1 -> Sum/1
  Sum/1 -> Sqrt/1
  Sqrt/1 -> DBR/1

== system Control_try_2/Team 1 Behaviour/Proximity_Finder_Ball3 ==
  In1 : Inport
  Demux : Demux  Outputs=2
  Sqrt : Sqrt  SaturateOnIntegerOverflow=on
  Square : Math  Operator=square  SaturateOnIntegerOverflow=on
  Square1 : Math  Operator=square  SaturateOnIntegerOverflow=on
  Sum : Sum
  DBR : Outport
  wires:
  In1/1 -> Demux/1
  Demux/1 -> Square/1
  Demux/2 -> Square1/1
  Square1/1 -> Sum/2
  Square/1 -> Sum/1
  Sum/1 -> Sqrt/1
  Sqrt/1 -> DBR/1

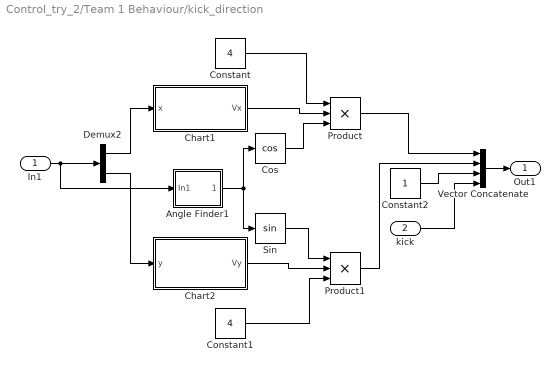
== system Control_try_2/Team 1 Behaviour/kick_direction ==
  In1 : Inport
  kick : Inport  Port=2
  Angle Finder1 : Subsystem
  Chart1 : Stateflow chart  TreatAsAtomicUnit=on
  Chart2 : Stateflow chart  TreatAsAtomicUnit=on
  Constant : Constant  Value=4
  Constant1 : Constant  Value=4
  Constant2 : Constant
  Cos : Trigonometry  Operator=cos
  Demux2 : Demux  Outputs=2
  Product : Product  Inputs=3
  Product1 : Product  Inputs=3
  Sin : Trigonometry
  Vector Concatenate : Concatenate  NumInputs=4
  Out1 : Outport
  wires:
  Demux2/2 -> Chart2/1(y)
  Demux2/1 -> Chart1/1(x)
  In1/1 -> Angle Finder1/1(In1), Demux2/1
  Chart1/1(Vx) -> Product/2
  Cos/1 -> Product/3
  Angle Finder1/1(angle) -> Cos/1, Sin/1
  Constant/1 -> Product/1
  Constant1/1 -> Product1/3
  Chart2/1(Vy) -> Product1/2
  Sin/1 -> Product1/1
  Product/1 -> Vector Concatenate/1
  Product1/1 -> Vector Concatenate/2
  Constant2/1 -> Vector Concatenate/3
  kick/1 -> Vector Concatenate/4
  Vector Concatenate/1 -> Out1/1

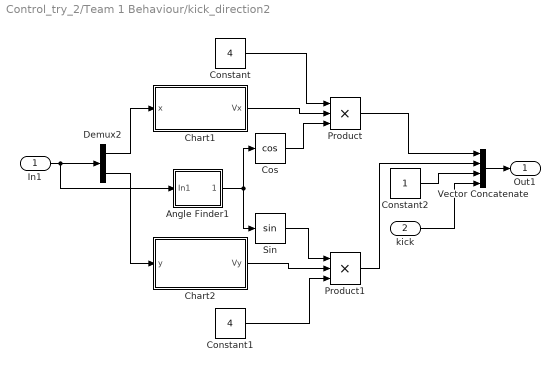
== system Control_try_2/Team 1 Behaviour/kick_direction2 ==
  In1 : Inport
  kick : Inport  Port=2
  Angle Finder1 : Subsystem
  Chart1 : Stateflow chart  TreatAsAtomicUnit=on
  Chart2 : Stateflow chart  TreatAsAtomicUnit=on
  Constant : Constant  Value=4
  Constant1 : Constant  Value=4
  Constant2 : Constant
  Cos : Trigonometry  Operator=cos
  Demux2 : Demux  Outputs=2
  Product : Product  Inputs=3
  Product1 : Product  Inputs=3
  Sin : Trigonometry
  Vector Concatenate : Concatenate  NumInputs=4
  Out1 : Outport
  wires:
  Demux2/2 -> Chart2/1(y)
  Demux2/1 -> Chart1/1(x)
  In1/1 -> Angle Finder1/1(In1), Demux2/1
  Chart1/1(Vx) -> Product/2
  Cos/1 -> Product/3
  Angle Finder1/1(angle) -> Cos/1, Sin/1
  Constant/1 -> Product/1
  Constant1/1 -> Product1/3
  Chart2/1(Vy) -> Product1/2
  Sin/1 -> Product1/1
  Product/1 -> Vector Concatenate/1
  Product1/1 -> Vector Concatenate/2
  Constant2/1 -> Vector Concatenate/3
  kick/1 -> Vector Concatenate/4
  Vector Concatenate/1 -> Out1/1

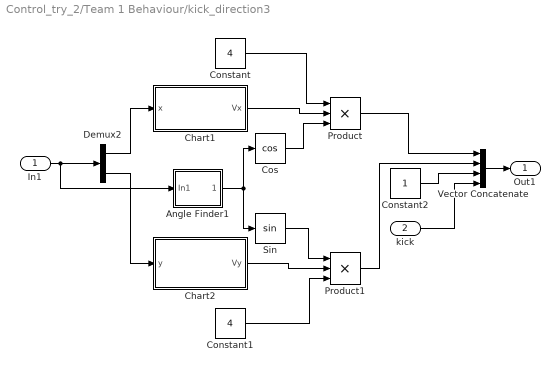
== system Control_try_2/Team 1 Behaviour/kick_direction3 ==
  In1 : Inport
  kick : Inport  Port=2
  Angle Finder1 : Subsystem
  Chart1 : Stateflow chart  TreatAsAtomicUnit=on
  Chart2 : Stateflow chart  TreatAsAtomicUnit=on
  Constant : Constant  Value=4
  Constant1 : Constant  Value=4
  Constant2 : Constant
  Cos : Trigonometry  Operator=cos
  Demux2 : Demux  Outputs=2
  Product : Product  Inputs=3
  Product1 : Product  Inputs=3
  Sin : Trigonometry
  Vector Concatenate : Concatenate  NumInputs=4
  Out1 : Outport
  wires:
  Demux2/2 -> Chart2/1(y)
  Demux2/1 -> Chart1/1(x)
  In1/1 -> Angle Finder1/1(In1), Demux2/1
  Chart1/1(Vx) -> Product/2
  Cos/1 -> Product/3
  Angle Finder1/1(angle) -> Cos/1, Sin/1
  Constant/1 -> Product/1
  Constant1/1 -> Product1/3
  Chart2/1(Vy) -> Product1/2
  Sin/1 -> Product1/1
  Product/1 -> Vector Concatenate/1
  Product1/1 -> Vector Concatenate/2
  Constant2/1 -> Vector Concatenate/3
  kick/1 -> Vector Concatenate/4
  Vector Concatenate/1 -> Out1/1

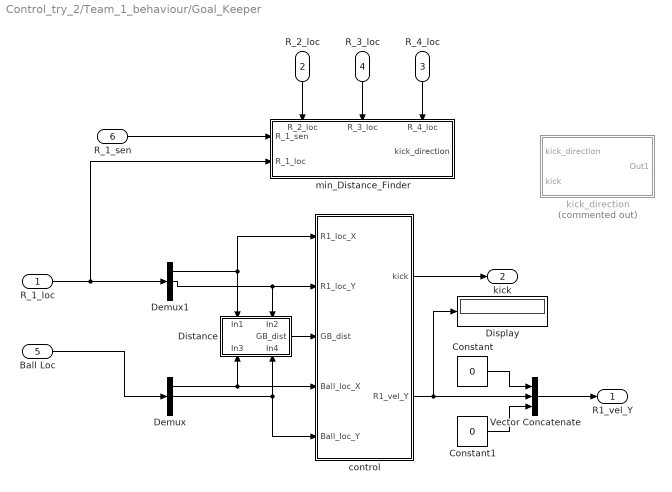
== system Control_try_2/Team_1_behaviour/Goal_Keeper ==
  R_1_loc : Inport
  R_2_loc : Inport  Port=2
  R_4_loc : Inport  Port=3
  R_3_loc : Inport  Port=4
  Ball Loc : Inport  Port=5
  R_1_sen : Inport  Port=6
  Constant : Constant  Value=0
  Constant1 : Constant  Value=0
  Demux : Demux  Outputs=3
  Demux1 : Demux  Outputs=3
  Display : Display
  Distance : Subsystem
      settings: PortSchema="{\"entries\":[{\"content\":{\"sides\":[{\"content\":{\"connectorIds\":[]},\"type\":\"ConnectorPlacement.EquallySpacedRectSide\",\"uuid\":\"931fdb8b-3711-4e7f-9cbc-53e0dea53fca\"},{\"content\":{\"connectorIds\":[\"Out1\"],\"side\":\"RIGHT\"},\"type\":\"ConnectorPlacement.EquallySpacedRectSide\",\"uuid\":\"ee0c7800-c700-48d1-aa4f-dd4a30624bbc\"},{\"content\":{\"connectorIds\":[\"In1\",\"In2\"],\"side\":\"TOP\"},\"type\":\"ConnectorPlacement.EquallySpacedRectSide\",\"uuid\":\"9579cc4b-8b33-4755-9564-e19cfe104d2b\"},{\"content\":{\"connectorIds\":[\"In3\",\"In4\"],\"side\":\"BOTTOM\"},\"type\":\"ConnectorPlacement.EquallySpacedRectSide\",\"uuid\":\"3469c1a3-363b-4534-8624-9a42e1898f6f\"}]},\"type\":\"ConnectorPlacement.EquallySpacedConnector\",\"uuid\":\"efd995f2-e999-4310-9f3f-88c38333e880\"}],\"packageUris\":[\"http://schema.mathworks.com/mf0/Connector/R2020b\"],\"version\":\"1.0\"}"
  Vector Concatenate : Concatenate  NumInputs=3
  control : Stateflow chart  TreatAsAtomicUnit=on
      settings: PortSchema="{\"entries\":[{\"content\":{\"sides\":[{\"content\":{\"connectorIds\":[\"In1\",\"In4\",\"In3\",\"In2\",\"In5\"]},\"type\":\"ConnectorPlacement.EquallySpacedRectSide\",\"uuid\":\"fa0fd246-e6b9-4dd4-94af-e6e1e45d6f7d\"},{\"content\":{\"connectorIds\":[\"Out1\",\"Out2\"],\"side\":\"RIGHT\"},\"type\":\"ConnectorPlacement.EquallySpacedRectSide\",\"uuid\":\"3f196244-96d1-41e4-aa84-a415e0f99109\"},{\"content\":{\"connectorIds\":[],\"side\":\"TOP\"},\"type\":\"ConnectorPlacement.EquallySpacedRectSide\",\"uuid\":\"731ebc3a-62ab-4275-8d10-19257bb8fb52\"}]},\"type\":\"ConnectorPlacement.EquallySpacedConnector\",\"uuid\":\"dccf28de-3df1-4952-8544-1d4b47a347e5\"}],\"packageUris\":[\"http://schema.mathworks.com/mf0/Connector/R2020b\"],\"version\":\"1.0\"}"
  kick_direction : Subsystem  Commented=on
  min_Distance_Finder : Subsystem
      settings: PortSchema="{\"entries\":[{\"content\":{\"sides\":[{\"content\":{\"connectorIds\":[\"In1\",\"In2\"]},\"type\":\"ConnectorPlacement.EquallySpacedRectSide\",\"uuid\":\"45cf91c7-7d38-4a19-bf35-d1d31095287a\"},{\"content\":{\"connectorIds\":[\"Out1\"],\"side\":\"RIGHT\"},\"type\":\"ConnectorPlacement.EquallySpacedRectSide\",\"uuid\":\"645394ba-2e5d-4060-b61c-cc9330ee0038\"},{\"content\":{\"connectorIds\":[\"In3\",\"In4\",\"In5\"],\"side\":\"TOP\"},\"type\":\"ConnectorPlacement.EquallySpacedRectSide\",\"uuid\":\"4fc56b73-04ec-476f-b487-f0e593f708ad\"},{\"content\":{\"connectorIds\":[],\"side\":\"BOTTOM\"},\"type\":\"ConnectorPlacement.EquallySpacedRectSide\",\"uuid\":\"cd306436-fd63-4e79-88e6-7a63c0840ed7\"}]},\"type\":\"ConnectorPlacement.EquallySpacedConnector\",\"uuid\":\"5cf2ee04-00eb-490b-958c-5fb90b43d325\"}],\"packageUris\":[\"http://schema.mathworks.com/mf0/Connector/R2020b\"],\"version\":\"1.0\"}"
  R1_vel_Y : Outport
  kick : Outport  Port=2
  wires:
  Ball Loc/1 -> Demux/1
  Demux/2 -> control/5(Ball_loc_Y), Distance/4(In4)
  R_1_loc/1 -> Demux1/1, min_Distance_Finder/2(R_1_loc)
  Demux1/2 -> control/4(R1_loc_Y), Distance/2(In2)
  Demux1/1 -> control/1(R1_loc_X), Distance/1(In1)
  R_2_loc/1 -> min_Distance_Finder/3(R_2_loc)
  R_3_loc/1 -> min_Distance_Finder/4(R_3_loc)
  R_4_loc/1 -> min_Distance_Finder/5(R_4_loc)
  R_1_sen/1 -> min_Distance_Finder/1(R_1_sen)
  Demux/1 -> control/2(Ball_loc_X), Distance/3(In3)
  control/2(R1_vel_Y) -> Vector Concatenate/2, Display/1
  Distance/1(GB_dist) -> control/3(GB_dist)
  Vector Concatenate/1 -> R1_vel_Y/1
  Constant/1 -> Vector Concatenate/1
  Constant1/1 -> Vector Concatenate/3
  control/1(kick) -> kick/1

== system Control_try_2/Team_1_behaviour/Goal_Keeper2 ==
  R_1_loc : Inport
  R_2_loc : Inport  Port=2
  R_4_loc : Inport  Port=3
  R_3_loc : Inport  Port=4
  Ball Loc : Inport  Port=5
  R_3_sen : Inport  Port=6
  Out1 : Outport
  Out2 : Outport  Port=2

== system Control_try_2/Team_1_behaviour/Goal_Keeper3 ==
  R_1_loc : Inport
  R_2_loc : Inport  Port=2
  R_4_loc : Inport  Port=3
  R_3_loc : Inport  Port=4
  Ball Loc : Inport  Port=5
  R_4_sen : Inport  Port=6
  Out1 : Outport
  Out2 : Outport  Port=2

== system Control_try_2/Team_1_behaviour/Roobot_2 ==
  R_1_loc : Inport
  R_2_loc : Inport  Port=2
  R_4_loc : Inport  Port=3
  R_3_loc : Inport  Port=4
  Ball Loc : Inport  Port=5
  R_2_sen : Inport  Port=6
  Out1 : Outport
  Out2 : Outport  Port=2

== system Control_try_2/Team 1 Behaviour/kick_direction/Angle Finder1 ==
  In1 : Inport
  Abs : Abs
  Atan : Trigonometry  Operator=atan
  Demux : Demux  Outputs=2
  Divide : Product  Inputs=/*
  angle : Outport
  wires:
  Divide/1 -> Atan/1
  Demux/2 -> Divide/2
  Demux/1 -> Divide/1
  Atan/1 -> Abs/1
  Abs/1 -> angle/1
  In1/1 -> Demux/1

== system Control_try_2/Team 1 Behaviour/kick_direction2/Angle Finder1 ==
  In1 : Inport
  Abs : Abs
  Atan : Trigonometry  Operator=atan
  Demux : Demux  Outputs=2
  Divide : Product  Inputs=/*
  angle : Outport
  wires:
  Divide/1 -> Atan/1
  Demux/2 -> Divide/2
  Demux/1 -> Divide/1
  Atan/1 -> Abs/1
  Abs/1 -> angle/1
  In1/1 -> Demux/1

== system Control_try_2/Team 1 Behaviour/kick_direction3/Angle Finder1 ==
  In1 : Inport
  Abs : Abs
  Atan : Trigonometry  Operator=atan
  Demux : Demux  Outputs=2
  Divide : Product  Inputs=/*
  angle : Outport
  wires:
  Divide/1 -> Atan/1
  Demux/2 -> Divide/2
  Demux/1 -> Divide/1
  Atan/1 -> Abs/1
  Abs/1 -> angle/1
  In1/1 -> Demux/1

== system Control_try_2/Team_1_behaviour/Goal_Keeper/Distance ==
  In1 : Inport
  In2 : Inport  Port=2
  In3 : Inport  Port=3
  In4 : Inport  Port=4
  Square : Math  Operator=square  SaturateOnIntegerOverflow=on
  Square Root : Sqrt  SaturateOnIntegerOverflow=on
  Square1 : Math  Operator=square  SaturateOnIntegerOverflow=on
  Sum : Sum  Inputs=|+-
  Sum1 : Sum  Inputs=|+-
  Sum2 : Sum  Inputs=|++
  GB_dist : Outport
  wires:
  Square1/1 -> Sum2/2
  Sum2/1 -> Square Root/1
  Square/1 -> Sum2/1
  Sum1/1 -> Square1/1
  Sum/1 -> Square/1
  In1/1 -> Sum/1
  In3/1 -> Sum/2
  In2/1 -> Sum1/1
  In4/1 -> Sum1/2
  Square Root/1 -> GB_dist/1

== system Control_try_2/Team_1_behaviour/Goal_Keeper/kick_direction ==
  kick_direction : Inport
  kick : Inport  Port=2
  Angle Finder1 : Subsystem
  Chart1 : Stateflow chart  TreatAsAtomicUnit=on
  Chart2 : Stateflow chart  TreatAsAtomicUnit=on
  Constant : Constant  Value=4
  Constant1 : Constant  Value=4
  Constant2 : Constant
  Cos : Trigonometry  Operator=cos
  Demux2 : Demux  Outputs=2
  Product : Product  Inputs=3
  Product1 : Product  Inputs=3
  Sin : Trigonometry
  Vector Concatenate : Concatenate  NumInputs=4
  Out1 : Outport
  wires:
  Demux2/2 -> Chart2/1(y)
  Demux2/1 -> Chart1/1(x)
  kick_direction/1 -> Angle Finder1/1(In1), Demux2/1
  Chart1/1(Vx) -> Product/2
  Cos/1 -> Product/3
  Angle Finder1/1(angle) -> Cos/1, Sin/1
  Constant/1 -> Product/1
  Constant1/1 -> Product1/3
  Chart2/1(Vy) -> Product1/2
  Sin/1 -> Product1/1
  Product/1 -> Vector Concatenate/1
  Product1/1 -> Vector Concatenate/2
  Constant2/1 -> Vector Concatenate/3
  kick/1 -> Vector Concatenate/4
  Vector Concatenate/1 -> Out1/1
